simulink model "PhaseII_opalrt_NoProtection"  (Simulink 8.8)
settings: Solver=ode3  StartTime=0.0  StopTime=inf  FixedStep=Ts  RelTol=1e-5  EnableMultiTasking=on
PostLoadFcn:
  | %BESS ctrl
  | Kpf=0.005*3*12;
  | Kif=5*6;
  | 
  | Kpf1=0.005*3*12;
  | Kif1=5*6;
  | Kp_v=0.016*15*35;
  | Ki_v=12*25;
  | 
  | Kp_v1=0.016*15*35;
  | Ki_v1=12*25;
  | 
  | Vabc_B=12.47e3;
  | Vdc_ref=Vabc_B*2;
  | Kpwm=sqrt(2)*Vabc_B/Vdc_ref;
  | ZB=Vabc_B^2/1e6;
  | R=0.005*ZB;
  | Ibasefull=673/2*sqrt(2);
  | 
  | 
  | Ts_Control=1e-4;
  | ts=0.05;
  | delay=0.2;
  | offset=10e3;
  | t_plan=60;
  | t_monitor=.2;
  | t_mon=t_monitor;
  | scalingfactor=1;
  | x=0.5;
  | n=6;
  | %t_plan=1/15;
  | %t_monitor=10/900;
  | %t_mon=10/900;
  | 
  | %t_plan=1/5;
  | %t_monitor=10/300;
  | %t_mon=10/300;
  | %scalingfactor=1/300;
  | 
  | f0=60;
  | 
  | Pabc_B=1e6;
  | Iabc_B=Pabc_B*sqrt(2/3)/Vabc_B;  % pk value
  | Imax_1=2.5;
  | Ptrans_B=Pabc_B*200;
  | 
  | Vdc_ref=Vabc_B*2;
  | 
  | ZB=Vabc_B^2/Pabc_B;
  | L=0.1*ZB/2/pi/60;
  | R=0.1*ZB;
  | C=1/(4*pi^2*(2e3)^2*L);
  | 
  | LL=0.005*ZB/2/pi/60;
  | RR=0.005*ZB;
  | 
  | RC=0.02;
  | 
  | %%% Initial SOC %%%%
  | SOC_ini_BESS1=0.5;
  | ... (+223 lines)
InitFcn:
  | %BESS ctrl
  | Kpf=0.005*3*12;
  | Kif=5*6;
  | 
  | Kpf1=0.005*3*12;
  | Kif1=5*6;
  | Kp_v=0.016*15*35;
  | Ki_v=12*25;
  | 
  | Kp_v1=0.016*15*35;
  | Ki_v1=12*25;
  | 
  | Vabc_B=12.47e3;
  | Vdc_ref=Vabc_B*2;
  | Kpwm=sqrt(2)*Vabc_B/Vdc_ref;
  | ZB=Vabc_B^2/1e6;
  | R=0.005*ZB;
  | Ibasefull=673/2*sqrt(2);
  | 
  | 
  | Ts_Control=1e-4;
  | ts=0.05;
  | delay=0.2;
  | offset=10e3;
  | t_plan=60;
  | t_monitor=.2;
  | t_mon=t_monitor;
  | scalingfactor=1;
  | x=0.5;
  | n=6;
  | %t_plan=1/15;
  | %t_monitor=10/900;
  | %t_mon=10/900;
  | 
  | %t_plan=1/5;
  | %t_monitor=10/300;
  | %t_mon=10/300;
  | %scalingfactor=1/300;
  | 
  | f0=60;
  | 
  | Pabc_B=1e6;
  | Iabc_B=Pabc_B*sqrt(2/3)/Vabc_B;  % pk value
  | Imax_1=2.5;
  | Ptrans_B=Pabc_B*200;
  | 
  | Vdc_ref=Vabc_B*2;
  | 
  | ZB=Vabc_B^2/Pabc_B;
  | L=0.1*ZB/2/pi/60;
  | R=0.1*ZB;
  | C=1/(4*pi^2*(2e3)^2*L);
  | 
  | LL=0.005*ZB/2/pi/60;
  | RR=0.005*ZB;
  | 
  | RC=0.02;
  | 
  | %%% Initial SOC %%%%
  | SOC_ini_BESS1=0.5;
  | ... (+223 lines)
undefined symbols (not defined in the file): D1, Delta, DiscIntNeverNeededParam, Left, PG2ref, type, V
libraries: powerlib x220, powerlib_meascontrol x82, dspstat3 x54, dsparch4 x43, dspswit3 x24, simulink x19, simulink_extras x12, powerlib_extras x11, ssn_lib x7, artemis x6, rtlab x5, rtio_generic_dnp3 x5
(part 6 of 9)

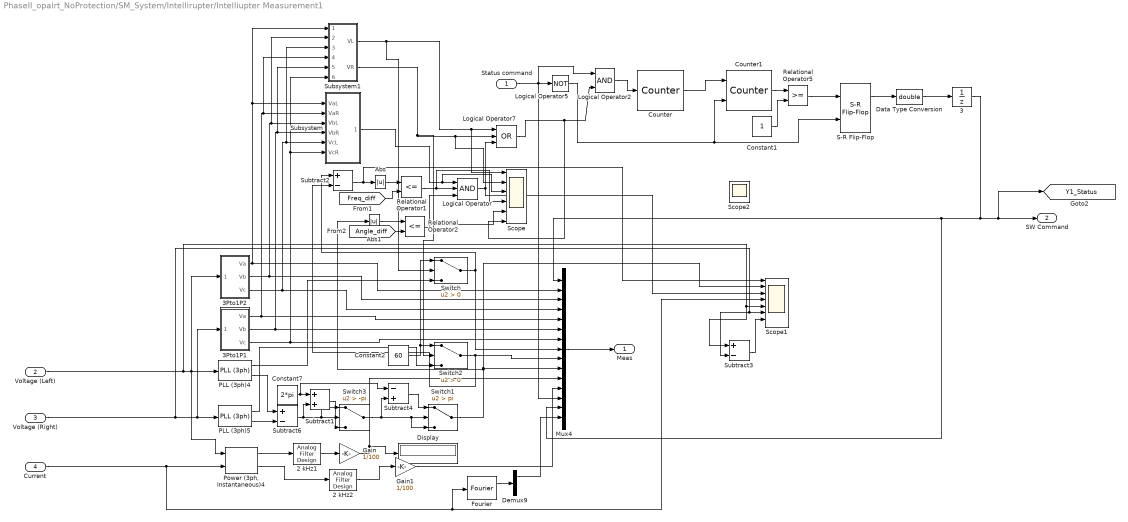
== system PhaseII_opalrt_NoProtection/SM_System/Intellirupter/Intelliupter Measurement1 ==
  Status command : Inport
  Voltage (Left) : Inport  Port=2
  Voltage (Right) : Inport  Port=3
  Current : Inport  Port=4
  "   3" : UnitDelay  SampleTime=Ts
  2 kHz1 : dsparch4/Analog Filter Design  method=Butterworth  filttype=Lowpass  N=2  Wlo=2*pi*5  Whi=80  Rp=2  Rs=40
  2 kHz2 : dsparch4/Analog Filter Design  method=Butterworth  filttype=Lowpass  N=2  Wlo=2*pi*5  Whi=80  Rp=2  Rs=40
  3Pto1P1 : Subsystem
  3Pto1P2 : Subsystem
  Abs : Abs
  Abs1 : Abs
  Constant1 : Constant
  Constant2 : Constant  Value=60
  Constant7 : Constant  Value=2*pi
  Counter : dspswit3/Counter  Direction=Up  CountEvent=Non-zero sample  CounterSize=User defined  MaxCount=10000  InitialCount=0  Output=Hit  HitValue=2000  ResetInput=off  SamplesPerFrame=1  Ts=1  CntDtype=double  HitDtype=Logical
  Counter1 : dspswit3/Counter  Direction=Up  CountEvent=Non-zero sample  CounterSize=User defined  MaxCount=255  InitialCount=0  Output=Count  HitValue=50  ResetInput=on  SamplesPerFrame=1  Ts=1  CntDtype=double  HitDtype=Logical
  Data Type Conversion : DataTypeConversion  OutDataTypeStr=double
  Demux9 : Demux  Outputs=3
  Display : Display
  Fourier : powerlib_meascontrol/Measurements/Fourier  Freq=60  n=1  InInit=[0, 0]  Ts=0
  Gain : Gain  Gain=1/100
  Gain1 : Gain  Gain=1/100
  Logical Operator : Logic  Inputs=3  AllPortsSameDT=off  OutDataTypeStr=boolean
  Logical Operator2 : Logic  AllPortsSameDT=off  OutDataTypeStr=boolean
  Logical Operator5 : Logic  Operator=NOT  AllPortsSameDT=off  OutDataTypeStr=boolean
  Logical Operator7 : Logic  Operator=OR  Inputs=3  AllPortsSameDT=off
  Mux4 : Mux  Inputs=15
  PLL (3ph)4 : powerlib_meascontrol/PLL/PLL (3ph)  Fmin=45  Par_Init=[0, 60]  ParK=[180, 3200, 1]  TcD=1e-4  MaxRateChangeFreq=12  FilterCutOffFreq=25  Ts=0  AGC=on
  PLL (3ph)5 : powerlib_meascontrol/PLL/PLL (3ph)  Fmin=45  Par_Init=[0, 60]  ParK=[180, 3200, 1]  TcD=1e-4  MaxRateChangeFreq=12  FilterCutOffFreq=25  Ts=0  AGC=on
  "Power (3ph, Instantaneous)4" : powerlib_meascontrol/Measurements/Power (3ph, Instantaneous)
  Relational Operator1 : RelationalOperator  Operator=<=  OutDataTypeStr=boolean  RndMeth=Simplest
  Relational Operator2 : RelationalOperator  Operator=<=  OutDataTypeStr=boolean  RndMeth=Simplest
  Relational Operator5 : RelationalOperator  OutDataTypeStr=boolean  RndMeth=Nearest
  S-R Flip-Flop : simulink_extras/Flip Flops/S-R Flip-Flop  initial_condition=0
  Scope : Scope  NumInputPorts=6
  Scope1 : Scope  NumInputPorts=8
  Scope2 : Scope  NumInputPorts=4
  Subsystem : Subsystem
  Subsystem1 : Subsystem
  Subtract1 : Sum
  Subtract2 : Sum  Inputs=+-
  Subtract3 : Sum  Inputs=+-
  Subtract4 : Sum  Inputs=-+
  Subtract6 : Sum  Inputs=+-
  Switch : Switch  Criteria=u2 > Threshold
  Switch1 : Switch  Criteria=u2 > Threshold  Threshold=pi
  Switch2 : Switch  Criteria=u2 > Threshold
  Switch3 : Switch  Criteria=u2 > Threshold  Threshold=-pi
  Meas : Outport
  SW Command : Outport  Port=2
  tag scope: Y1_Status=global
  wires:
  Logical Operator5/1 -> Counter1/2, S-R Flip-Flop/2
  Demux9/1 -> Mux4/15
  Fourier/1 -> Demux9/1
  Current/1 -> "Power (3ph, Instantaneous)4"/2, Scope1/4, Fourier/1
  Voltage (Left)/1 -> 3Pto1P2/1(Vabc), PLL (3ph)4/1, "Power (3ph, Instantaneous)4"/1, Scope1/5, Subtract3/1
  Subtract1/1 -> Switch3/3
  Subtract3/1 -> Scope1/7
  Constant7/1 -> Subtract4/1, Subtract1/1
  Subtract6/1 -> Switch3/2, Switch3/1, Subtract1/2
  Voltage (Right)/1 -> 3Pto1P1/1(Vabc), PLL (3ph)5/1, Scope1/6, Subtract3/2
  Subsystem1/2(VR) -> Switch2/2, Scope/2, Logical Operator7/2
  Subsystem1/1(VL) -> Switch/2, Scope/1, Logical Operator7/1
  Subsystem/1(Vdiff) -> Scope/3, Logical Operator/1
  Counter1/1 -> Relational Operator5/1
  Counter/1 -> Counter1/1
  Constant1/1 -> Relational Operator5/2
  Logical Operator2/1 -> Counter/1
  "Power (3ph, Instantaneous)4"/1 -> 2 kHz1/1
  PLL (3ph)4/1 -> Switch/3
  3Pto1P1/3(Vc) -> Mux4/7, Subsystem/6(VcR), Subsystem1/6(VcR)
  3Pto1P1/2(Vb) -> Mux4/6, Subsystem/4(VbR), Subsystem1/5(VbR)
  3Pto1P1/1(Va) -> Subsystem/2(VaR), Subsystem1/4(VaR), Mux4/5
  3Pto1P2/3(Vc) -> Mux4/4, Subsystem/5(VcL), Subsystem1/3(VcL)
  3Pto1P2/2(Vb) -> Subsystem/3(VbL), Subsystem1/2(VbL), Mux4/3
  3Pto1P2/1(Va) -> Mux4/2, Subsystem/1(VaL), Subsystem1/1(VaL)
  PLL (3ph)4/2 -> Subtract6/1
  Mux4/1 -> Meas/1
  PLL (3ph)5/2 -> Subtract6/2
  Relational Operator1/1 -> Scope/4, Logical Operator/2
  Relational Operator2/1 -> Scope/5, Logical Operator/3
  Subtract2/1 -> Abs/1, Scope1/1
  [Freq_diff] -> Relational Operator1/2
  [Angle_diff] -> Relational Operator2/2
  Logical Operator/1 -> Logical Operator7/3, Scope1/3
  Status command/1 -> Logical Operator2/1, Mux4/13, Logical Operator5/1
  Logical Operator7/1 -> Scope/6, Logical Operator2/2
  "Power (3ph, Instantaneous)4"/2 -> 2 kHz2/1
  "   3"/1 -> Mux4/1, Mux4/14, [Y1_Status], SW Command/1
  2 kHz1/1 -> Gain/1
  2 kHz2/1 -> Gain1/1
  Gain/1 -> Mux4/11, Display/1
  Gain1/1 -> Mux4/12
  S-R Flip-Flop/1 -> Data Type Conversion/1
  Relational Operator5/1 -> S-R Flip-Flop/1
  Data Type Conversion/1 -> "   3"/1
  Switch1/1 -> Scope1/2, Mux4/10, Abs1/1
  Subtract4/1 -> Switch1/1
  Switch3/1 -> Subtract4/2, Switch1/3, Switch1/2
  Abs/1 -> Relational Operator1/1
  Abs1/1 -> Relational Operator2/1
  Switch/1 -> Mux4/8, Subtract2/1
  Switch2/1 -> Subtract2/2, Mux4/9
  PLL (3ph)5/1 -> Switch2/3
  Constant2/1 -> Switch/1, Switch2/1

== system PhaseII_opalrt_NoProtection/SM_System/Intellirupter/Intelliupter Measurement2 ==
  Status command : Inport
  Voltage (Left) : Inport  Port=2
  Voltage (Right) : Inport  Port=3
  Current : Inport  Port=4
  "   3" : UnitDelay  SampleTime=Ts
  2 kHz1 : dsparch4/Analog Filter Design  method=Butterworth  filttype=Lowpass  N=2  Wlo=2*pi*5  Whi=80  Rp=2  Rs=40
  2 kHz2 : dsparch4/Analog Filter Design  method=Butterworth  filttype=Lowpass  N=2  Wlo=2*pi*5  Whi=80  Rp=2  Rs=40
  3Pto1P1 : Subsystem
  3Pto1P2 : Subsystem
  Abs : Abs
  Abs1 : Abs
  Constant1 : Constant
  Constant2 : Constant  Value=60
  Constant7 : Constant  Value=2*pi
  Counter : dspswit3/Counter  Direction=Up  CountEvent=Non-zero sample  CounterSize=User defined  MaxCount=10000  InitialCount=0  Output=Hit  HitValue=2000  ResetInput=off  SamplesPerFrame=1  Ts=1  CntDtype=double  HitDtype=Logical
  Counter1 : dspswit3/Counter  Direction=Up  CountEvent=Non-zero sample  CounterSize=User defined  MaxCount=255  InitialCount=0  Output=Count  HitValue=50  ResetInput=on  SamplesPerFrame=1  Ts=1  CntDtype=double  HitDtype=Logical
  Data Type Conversion : DataTypeConversion  OutDataTypeStr=double
  Demux9 : Demux  Outputs=3
  Display : Display
  Fourier : powerlib_meascontrol/Measurements/Fourier  Freq=60  n=1  InInit=[0, 0]  Ts=0
  Gain : Gain  Gain=1/100
  Gain1 : Gain  Gain=1/100
  Logical Operator : Logic  Inputs=3  AllPortsSameDT=off  OutDataTypeStr=boolean
  Logical Operator2 : Logic  AllPortsSameDT=off  OutDataTypeStr=boolean
  Logical Operator5 : Logic  Operator=NOT  AllPortsSameDT=off  OutDataTypeStr=boolean
  Logical Operator7 : Logic  Operator=OR  Inputs=3  AllPortsSameDT=off
  Mux4 : Mux  Inputs=15
  PLL (3ph)4 : powerlib_meascontrol/PLL/PLL (3ph)  Fmin=45  Par_Init=[0, 60]  ParK=[180, 3200, 1]  TcD=1e-4  MaxRateChangeFreq=12  FilterCutOffFreq=25  Ts=0  AGC=on
  PLL (3ph)5 : powerlib_meascontrol/PLL/PLL (3ph)  Fmin=45  Par_Init=[0, 60]  ParK=[180, 3200, 1]  TcD=1e-4  MaxRateChangeFreq=12  FilterCutOffFreq=25  Ts=0  AGC=on
  "Power (3ph, Instantaneous)4" : powerlib_meascontrol/Measurements/Power (3ph, Instantaneous)
  Relational Operator1 : RelationalOperator  Operator=<=  OutDataTypeStr=boolean  RndMeth=Simplest
  Relational Operator2 : RelationalOperator  Operator=<=  OutDataTypeStr=boolean  RndMeth=Simplest
  Relational Operator5 : RelationalOperator  OutDataTypeStr=boolean  RndMeth=Nearest
  S-R Flip-Flop : simulink_extras/Flip Flops/S-R Flip-Flop  initial_condition=0
  Scope1 : Scope  NumInputPorts=8
  Subsystem : Subsystem
  Subsystem1 : Subsystem
  Subtract1 : Sum
  Subtract2 : Sum  Inputs=+-
  Subtract3 : Sum  Inputs=+-
  Subtract4 : Sum  Inputs=-+
  Subtract6 : Sum  Inputs=+-
  Switch : Switch  Criteria=u2 > Threshold
  Switch1 : Switch  Criteria=u2 > Threshold  Threshold=pi
  Switch2 : Switch  Criteria=u2 > Threshold
  Switch3 : Switch  Criteria=u2 > Threshold  Threshold=-pi
  Meas : Outport
  SW Command : Outport  Port=2
  tag scope: Y2_Status=global
  wires:
  Logical Operator5/1 -> Counter1/2, S-R Flip-Flop/2
  "   3"/1 -> SW Command/1, [Y2_Status], Mux4/1, Mux4/14
  Demux9/1 -> Mux4/15
  Fourier/1 -> Demux9/1
  Current/1 -> "Power (3ph, Instantaneous)4"/2, Scope1/4, Fourier/1
  Voltage (Left)/1 -> 3Pto1P2/1(Vabc), PLL (3ph)4/1, "Power (3ph, Instantaneous)4"/1, Scope1/5, Subtract3/1
  Subtract1/1 -> Switch3/3
  Subtract3/1 -> Scope1/7
  Constant7/1 -> Subtract4/1, Subtract1/1
  Subtract6/1 -> Switch3/2, Switch3/1, Subtract1/2
  Voltage (Right)/1 -> 3Pto1P1/1(Vabc), PLL (3ph)5/1, Scope1/6, Subtract3/2
  Subsystem1/2(VR) -> Switch2/2, Logical Operator7/2
  Subsystem1/1(VL) -> Switch/2, Logical Operator7/1
  Subsystem/1(Vdiff) -> Logical Operator/1
  Counter1/1 -> Relational Operator5/1
  Counter/1 -> Counter1/1
  Constant1/1 -> Relational Operator5/2
  Logical Operator2/1 -> Counter/1
  "Power (3ph, Instantaneous)4"/1 -> 2 kHz1/1
  3Pto1P1/3(Vc) -> Mux4/7, Subsystem/6(VcR), Subsystem1/6(VcR)
  3Pto1P1/2(Vb) -> Mux4/6, Subsystem/4(VbR), Subsystem1/5(VbR)
  3Pto1P1/1(Va) -> Subsystem/2(VaR), Subsystem1/4(VaR), Mux4/5
  3Pto1P2/3(Vc) -> Mux4/4, Subsystem/5(VcL), Subsystem1/3(VcL)
  3Pto1P2/2(Vb) -> Subsystem/3(VbL), Subsystem1/2(VbL), Mux4/3
  3Pto1P2/1(Va) -> Mux4/2, Subsystem/1(VaL), Subsystem1/1(VaL)
  PLL (3ph)4/2 -> Subtract6/1
  Mux4/1 -> Meas/1
  PLL (3ph)5/2 -> Subtract6/2
  Relational Operator1/1 -> Logical Operator/2
  Relational Operator2/1 -> Logical Operator/3
  Subtract2/1 -> Abs/1, Scope1/1
  [Freq_diff] -> Relational Operator1/2
  [Angle_diff] -> Relational Operator2/2
  Logical Operator/1 -> Logical Operator7/3, Scope1/3
  Status command/1 -> Logical Operator2/1, Mux4/13, Logical Operator5/1
  Logical Operator7/1 -> Logical Operator2/2
  "Power (3ph, Instantaneous)4"/2 -> 2 kHz2/1
  2 kHz1/1 -> Gain/1
  2 kHz2/1 -> Gain1/1
  Gain/1 -> Mux4/11, Display/1
  Gain1/1 -> Mux4/12
  S-R Flip-Flop/1 -> Data Type Conversion/1
  Relational Operator5/1 -> S-R Flip-Flop/1
  Data Type Conversion/1 -> "   3"/1
  Switch1/1 -> Scope1/2, Mux4/10, Abs1/1
  Subtract4/1 -> Switch1/1
  Switch3/1 -> Subtract4/2, Switch1/3, Switch1/2
  Abs/1 -> Relational Operator1/1
  Abs1/1 -> Relational Operator2/1
  Switch/1 -> Subtract2/1, Mux4/8
  Switch2/1 -> Subtract2/2, Mux4/9
  PLL (3ph)4/1 -> Switch/3
  PLL (3ph)5/1 -> Switch2/3
  Constant2/1 -> Switch/1, Switch2/1

== system PhaseII_opalrt_NoProtection/SM_System/Intellirupter/Intelliupter Measurement3 ==
  Status command : Inport
  Voltage (Left) : Inport  Port=2
  Voltage (Right) : Inport  Port=3
  Current : Inport  Port=4
  "   3" : UnitDelay  SampleTime=Ts
  2 kHz1 : dsparch4/Analog Filter Design  method=Butterworth  filttype=Lowpass  N=2  Wlo=2*pi*5  Whi=80  Rp=2  Rs=40
  2 kHz2 : dsparch4/Analog Filter Design  method=Butterworth  filttype=Lowpass  N=2  Wlo=2*pi*5  Whi=80  Rp=2  Rs=40
  3Pto1P1 : Subsystem
  3Pto1P2 : Subsystem
  Abs : Abs
  Abs1 : Abs
  Constant1 : Constant
  Constant2 : Constant  Value=60
  Constant7 : Constant  Value=2*pi
  Counter : dspswit3/Counter  Direction=Up  CountEvent=Non-zero sample  CounterSize=User defined  MaxCount=10000  InitialCount=0  Output=Hit  HitValue=2000  ResetInput=off  SamplesPerFrame=1  Ts=1  CntDtype=double  HitDtype=Logical
  Counter1 : dspswit3/Counter  Direction=Up  CountEvent=Non-zero sample  CounterSize=User defined  MaxCount=255  InitialCount=0  Output=Count  HitValue=50  ResetInput=on  SamplesPerFrame=1  Ts=1  CntDtype=double  HitDtype=Logical
  Data Type Conversion : DataTypeConversion  OutDataTypeStr=double
  Demux9 : Demux  Outputs=3
  Display : Display
  Fourier : powerlib_meascontrol/Measurements/Fourier  Freq=60  n=1  InInit=[0, 0]  Ts=0
  Gain : Gain  Gain=1/100
  Gain1 : Gain  Gain=1/100
  Logical Operator : Logic  Inputs=3  AllPortsSameDT=off  OutDataTypeStr=boolean
  Logical Operator2 : Logic  AllPortsSameDT=off  OutDataTypeStr=boolean
  Logical Operator5 : Logic  Operator=NOT  AllPortsSameDT=off  OutDataTypeStr=boolean
  Logical Operator7 : Logic  Operator=OR  Inputs=3  AllPortsSameDT=off
  Mux4 : Mux  Inputs=15
  PLL (3ph)4 : powerlib_meascontrol/PLL/PLL (3ph)  Fmin=45  Par_Init=[0, 60]  ParK=[180, 3200, 1]  TcD=1e-4  MaxRateChangeFreq=12  FilterCutOffFreq=25  Ts=0  AGC=on
  PLL (3ph)5 : powerlib_meascontrol/PLL/PLL (3ph)  Fmin=45  Par_Init=[0, 60]  ParK=[180, 3200, 1]  TcD=1e-4  MaxRateChangeFreq=12  FilterCutOffFreq=25  Ts=0  AGC=on
  "Power (3ph, Instantaneous)4" : powerlib_meascontrol/Measurements/Power (3ph, Instantaneous)
  Relational Operator1 : RelationalOperator  Operator=<=  OutDataTypeStr=boolean  RndMeth=Simplest
  Relational Operator2 : RelationalOperator  Operator=<=  OutDataTypeStr=boolean  RndMeth=Simplest
  Relational Operator5 : RelationalOperator  OutDataTypeStr=boolean  RndMeth=Nearest
  S-R Flip-Flop : simulink_extras/Flip Flops/S-R Flip-Flop  initial_condition=0
  Scope1 : Scope  NumInputPorts=8
  Subsystem : Subsystem
  Subsystem1 : Subsystem
  Subtract1 : Sum
  Subtract2 : Sum  Inputs=+-
  Subtract3 : Sum  Inputs=+-
  Subtract4 : Sum  Inputs=-+
  Subtract6 : Sum  Inputs=+-
  Switch : Switch  Criteria=u2 > Threshold
  Switch1 : Switch  Criteria=u2 > Threshold  Threshold=pi
  Switch2 : Switch  Criteria=u2 > Threshold
  Switch3 : Switch  Criteria=u2 > Threshold  Threshold=-pi
  Meas : Outport
  SW Command : Outport  Port=2
  tag scope: Y3_Status=global
  wires:
  Logical Operator5/1 -> Counter1/2, S-R Flip-Flop/2
  "   3"/1 -> [Y3_Status], SW Command/1, Mux4/1, Mux4/14
  Demux9/1 -> Mux4/15
  Fourier/1 -> Demux9/1
  Current/1 -> "Power (3ph, Instantaneous)4"/2, Scope1/4, Fourier/1
  Voltage (Left)/1 -> 3Pto1P2/1(Vabc), PLL (3ph)4/1, "Power (3ph, Instantaneous)4"/1, Scope1/5, Subtract3/1
  Subtract1/1 -> Switch3/3
  Subtract3/1 -> Scope1/7
  Constant7/1 -> Subtract4/1, Subtract1/1
  Subtract6/1 -> Switch3/2, Switch3/1, Subtract1/2
  Voltage (Right)/1 -> 3Pto1P1/1(Vabc), PLL (3ph)5/1, Scope1/6, Subtract3/2
  Subsystem1/2(VR) -> Switch2/2, Logical Operator7/2
  Subsystem1/1(VL) -> Switch/2, Logical Operator7/1
  Subsystem/1(Vdiff) -> Logical Operator/1
  Counter1/1 -> Relational Operator5/1
  Counter/1 -> Counter1/1
  Constant1/1 -> Relational Operator5/2
  Logical Operator2/1 -> Counter/1
  "Power (3ph, Instantaneous)4"/1 -> 2 kHz1/1
  3Pto1P1/3(Vc) -> Mux4/7, Subsystem/6(VcR), Subsystem1/6(VcR)
  3Pto1P1/2(Vb) -> Mux4/6, Subsystem/4(VbR), Subsystem1/5(VbR)
  3Pto1P1/1(Va) -> Subsystem/2(VaR), Subsystem1/4(VaR), Mux4/5
  3Pto1P2/3(Vc) -> Mux4/4, Subsystem/5(VcL), Subsystem1/3(VcL)
  3Pto1P2/2(Vb) -> Subsystem/3(VbL), Subsystem1/2(VbL), Mux4/3
  3Pto1P2/1(Va) -> Mux4/2, Subsystem/1(VaL), Subsystem1/1(VaL)
  PLL (3ph)4/2 -> Subtract6/1
  Mux4/1 -> Meas/1
  PLL (3ph)5/2 -> Subtract6/2
  Relational Operator1/1 -> Logical Operator/2
  Relational Operator2/1 -> Logical Operator/3
  Subtract2/1 -> Abs/1, Scope1/1
  [Freq_diff] -> Relational Operator1/2
  [Angle_diff] -> Relational Operator2/2
  Logical Operator/1 -> Logical Operator7/3, Scope1/3
  Status command/1 -> Logical Operator2/1, Mux4/13, Logical Operator5/1
  Logical Operator7/1 -> Logical Operator2/2
  "Power (3ph, Instantaneous)4"/2 -> 2 kHz2/1
  2 kHz1/1 -> Gain/1
  2 kHz2/1 -> Gain1/1
  Gain/1 -> Mux4/11, Display/1
  Gain1/1 -> Mux4/12
  S-R Flip-Flop/1 -> Data Type Conversion/1
  Relational Operator5/1 -> S-R Flip-Flop/1
  Data Type Conversion/1 -> "   3"/1
  Switch1/1 -> Abs1/1, Scope1/2, Mux4/10
  Subtract4/1 -> Switch1/1
  Switch3/1 -> Subtract4/2, Switch1/3, Switch1/2
  Abs/1 -> Relational Operator1/1
  Abs1/1 -> Relational Operator2/1
  PLL (3ph)4/1 -> Switch/3
  PLL (3ph)5/1 -> Switch2/3
  Switch/1 -> Mux4/8, Subtract2/1
  Switch2/1 -> Subtract2/2, Mux4/9
  Constant2/1 -> Switch2/1, Switch/1

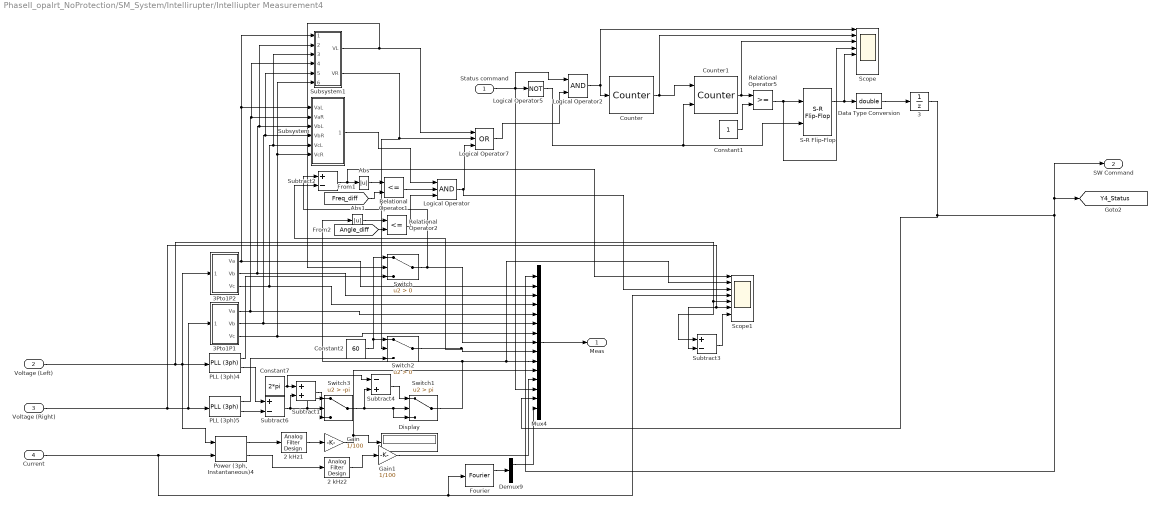
== system PhaseII_opalrt_NoProtection/SM_System/Intellirupter/Intelliupter Measurement4 ==
  Status command : Inport
  Voltage (Left) : Inport  Port=2
  Voltage (Right) : Inport  Port=3
  Current : Inport  Port=4
  "   3" : UnitDelay  SampleTime=Ts
  2 kHz1 : dsparch4/Analog Filter Design  method=Butterworth  filttype=Lowpass  N=2  Wlo=2*pi*5  Whi=80  Rp=2  Rs=40
  2 kHz2 : dsparch4/Analog Filter Design  method=Butterworth  filttype=Lowpass  N=2  Wlo=2*pi*5  Whi=80  Rp=2  Rs=40
  3Pto1P1 : Subsystem
  3Pto1P2 : Subsystem
  Abs : Abs
  Abs1 : Abs
  Constant1 : Constant
  Constant2 : Constant  Value=60
  Constant7 : Constant  Value=2*pi
  Counter : dspswit3/Counter  Direction=Up  CountEvent=Non-zero sample  CounterSize=User defined  MaxCount=10000  InitialCount=0  Output=Hit  HitValue=2000  ResetInput=off  SamplesPerFrame=1  Ts=1  CntDtype=double  HitDtype=Logical
  Counter1 : dspswit3/Counter  Direction=Up  CountEvent=Non-zero sample  CounterSize=User defined  MaxCount=255  InitialCount=0  Output=Count  HitValue=50  ResetInput=on  SamplesPerFrame=1  Ts=1  CntDtype=double  HitDtype=Logical
  Data Type Conversion : DataTypeConversion  OutDataTypeStr=double
  Demux9 : Demux  Outputs=3
  Display : Display
  Fourier : powerlib_meascontrol/Measurements/Fourier  Freq=60  n=1  InInit=[0, 0]  Ts=0
  Gain : Gain  Gain=1/100
  Gain1 : Gain  Gain=1/100
  Logical Operator : Logic  Inputs=3  AllPortsSameDT=off  OutDataTypeStr=boolean
  Logical Operator2 : Logic  AllPortsSameDT=off  OutDataTypeStr=boolean
  Logical Operator5 : Logic  Operator=NOT  AllPortsSameDT=off  OutDataTypeStr=boolean
  Logical Operator7 : Logic  Operator=OR  Inputs=3  AllPortsSameDT=off
  Mux4 : Mux  Inputs=15
  PLL (3ph)4 : powerlib_meascontrol/PLL/PLL (3ph)  Fmin=45  Par_Init=[0, 60]  ParK=[180, 3200, 1]  TcD=1e-4  MaxRateChangeFreq=12  FilterCutOffFreq=25  Ts=0  AGC=on
  PLL (3ph)5 : powerlib_meascontrol/PLL/PLL (3ph)  Fmin=45  Par_Init=[0, 60]  ParK=[180, 3200, 1]  TcD=1e-4  MaxRateChangeFreq=12  FilterCutOffFreq=25  Ts=0  AGC=on
  "Power (3ph, Instantaneous)4" : powerlib_meascontrol/Measurements/Power (3ph, Instantaneous)
  Relational Operator1 : RelationalOperator  Operator=<=  OutDataTypeStr=boolean  RndMeth=Simplest
  Relational Operator2 : RelationalOperator  Operator=<=  OutDataTypeStr=boolean  RndMeth=Simplest
  Relational Operator5 : RelationalOperator  OutDataTypeStr=boolean  RndMeth=Nearest
  S-R Flip-Flop : simulink_extras/Flip Flops/S-R Flip-Flop  initial_condition=0
  Scope : Scope  NumInputPorts=8
  Scope1 : Scope  NumInputPorts=8
  Subsystem : Subsystem
  Subsystem1 : Subsystem
  Subtract1 : Sum
  Subtract2 : Sum  Inputs=+-
  Subtract3 : Sum  Inputs=+-
  Subtract4 : Sum  Inputs=-+
  Subtract6 : Sum  Inputs=+-
  Switch : Switch  Criteria=u2 > Threshold
  Switch1 : Switch  Criteria=u2 > Threshold  Threshold=pi
  Switch2 : Switch  Criteria=u2 > Threshold
  Switch3 : Switch  Criteria=u2 > Threshold  Threshold=-pi
  Meas : Outport
  SW Command : Outport  Port=2
  tag scope: Y4_Status=global
  wires:
  Logical Operator5/1 -> Counter1/2, S-R Flip-Flop/2
  "   3"/1 -> Mux4/1, SW Command/1, [Y4_Status], Mux4/14
  Demux9/1 -> Mux4/15
  Fourier/1 -> Demux9/1
  Current/1 -> "Power (3ph, Instantaneous)4"/2, Scope1/4, Fourier/1
  Voltage (Left)/1 -> 3Pto1P2/1(Vabc), PLL (3ph)4/1, "Power (3ph, Instantaneous)4"/1, Scope1/5, Subtract3/1
  Subtract1/1 -> Switch3/3
  Subtract3/1 -> Scope1/7
  Constant7/1 -> Subtract4/1, Subtract1/1
  Subtract6/1 -> Switch3/2, Switch3/1, Subtract1/2
  Voltage (Right)/1 -> 3Pto1P1/1(Vabc), PLL (3ph)5/1, Scope1/6, Subtract3/2
  Subsystem1/2(VR) -> Switch2/2, Logical Operator7/2
  Subsystem1/1(VL) -> Switch/2, Logical Operator7/1
  Subsystem/1(Vdiff) -> Logical Operator/1
  Counter1/1 -> Relational Operator5/1, Scope/3
  Counter/1 -> Counter1/1, Scope/2
  Constant1/1 -> Relational Operator5/2
  Logical Operator2/1 -> Scope/1, Counter/1
  "Power (3ph, Instantaneous)4"/1 -> 2 kHz1/1
  3Pto1P1/3(Vc) -> Mux4/7, Subsystem/6(VcR), Subsystem1/6(VcR)
  3Pto1P1/2(Vb) -> Mux4/6, Subsystem/4(VbR), Subsystem1/5(VbR)
  3Pto1P1/1(Va) -> Subsystem/2(VaR), Subsystem1/4(VaR), Mux4/5
  3Pto1P2/3(Vc) -> Mux4/4, Subsystem/5(VcL), Subsystem1/3(VcL)
  3Pto1P2/2(Vb) -> Subsystem/3(VbL), Subsystem1/2(VbL), Mux4/3
  3Pto1P2/1(Va) -> Mux4/2, Subsystem/1(VaL), Subsystem1/1(VaL)
  PLL (3ph)4/2 -> Subtract6/1
  Mux4/1 -> Meas/1
  PLL (3ph)5/2 -> Subtract6/2
  Relational Operator1/1 -> Logical Operator/2
  Relational Operator2/1 -> Logical Operator/3
  Subtract2/1 -> Abs/1, Scope1/1
  [Freq_diff] -> Relational Operator1/2
  [Angle_diff] -> Relational Operator2/2
  Logical Operator/1 -> Logical Operator7/3, Scope1/3
  Status command/1 -> Logical Operator2/1, Mux4/13, Logical Operator5/1
  Logical Operator7/1 -> Logical Operator2/2
  "Power (3ph, Instantaneous)4"/2 -> 2 kHz2/1
  2 kHz1/1 -> Gain/1
  2 kHz2/1 -> Gain1/1
  Gain/1 -> Mux4/11, Display/1
  Gain1/1 -> Mux4/12
  S-R Flip-Flop/1 -> Data Type Conversion/1, Scope/5
  Relational Operator5/1 -> S-R Flip-Flop/1, Scope/4
  Data Type Conversion/1 -> "   3"/1
  Switch1/1 -> Scope1/2, Mux4/10, Abs1/1
  Subtract4/1 -> Switch1/1
  Switch3/1 -> Subtract4/2, Switch1/3, Switch1/2
  Abs/1 -> Relational Operator1/1
  Abs1/1 -> Relational Operator2/1
  Switch2/1 -> Subtract2/2, Mux4/9
  Switch/1 -> Mux4/8, Subtract2/1
  PLL (3ph)4/1 -> Switch/3
  PLL (3ph)5/1 -> Switch2/3
  Constant2/1 -> Switch/1, Switch2/1

== system PhaseII_opalrt_NoProtection/SM_System/Intellirupter/Intelliupter Measurement5 ==
  Status command : Inport
  Voltage (Left) : Inport  Port=2
  Voltage (Right) : Inport  Port=3
  Current : Inport  Port=4
  "   3" : UnitDelay  SampleTime=Ts
  2 kHz1 : dsparch4/Analog Filter Design  method=Butterworth  filttype=Lowpass  N=2  Wlo=2*pi*5  Whi=80  Rp=2  Rs=40
  2 kHz2 : dsparch4/Analog Filter Design  method=Butterworth  filttype=Lowpass  N=2  Wlo=2*pi*5  Whi=80  Rp=2  Rs=40
  3Pto1P1 : Subsystem
  3Pto1P2 : Subsystem
  Abs : Abs
  Abs1 : Abs
  Constant1 : Constant
  Constant2 : Constant  Value=60
  Constant7 : Constant  Value=2*pi
  Counter : dspswit3/Counter  Direction=Up  CountEvent=Non-zero sample  CounterSize=User defined  MaxCount=10000  InitialCount=0  Output=Hit  HitValue=2000  ResetInput=off  SamplesPerFrame=1  Ts=1  CntDtype=double  HitDtype=Logical
  Counter1 : dspswit3/Counter  Direction=Up  CountEvent=Non-zero sample  CounterSize=User defined  MaxCount=255  InitialCount=0  Output=Count  HitValue=50  ResetInput=on  SamplesPerFrame=1  Ts=1  CntDtype=double  HitDtype=Logical
  Data Type Conversion : DataTypeConversion  OutDataTypeStr=double
  Demux9 : Demux  Outputs=3
  Display : Display
  Fourier : powerlib_meascontrol/Measurements/Fourier  Freq=60  n=1  InInit=[0, 0]  Ts=0
  Gain : Gain  Gain=1/100
  Gain1 : Gain  Gain=1/100
  Logical Operator : Logic  Inputs=3  AllPortsSameDT=off  OutDataTypeStr=boolean
  Logical Operator2 : Logic  AllPortsSameDT=off  OutDataTypeStr=boolean
  Logical Operator5 : Logic  Operator=NOT  AllPortsSameDT=off  OutDataTypeStr=boolean
  Logical Operator7 : Logic  Operator=OR  Inputs=3  AllPortsSameDT=off
  Mux4 : Mux  Inputs=15
  PLL (3ph)4 : powerlib_meascontrol/PLL/PLL (3ph)  Fmin=45  Par_Init=[0, 60]  ParK=[180, 3200, 1]  TcD=1e-4  MaxRateChangeFreq=12  FilterCutOffFreq=25  Ts=0  AGC=on
  PLL (3ph)5 : powerlib_meascontrol/PLL/PLL (3ph)  Fmin=45  Par_Init=[0, 60]  ParK=[180, 3200, 1]  TcD=1e-4  MaxRateChangeFreq=12  FilterCutOffFreq=25  Ts=0  AGC=on
  "Power (3ph, Instantaneous)4" : powerlib_meascontrol/Measurements/Power (3ph, Instantaneous)
  Relational Operator1 : RelationalOperator  Operator=<=  OutDataTypeStr=boolean  RndMeth=Simplest
  Relational Operator2 : RelationalOperator  Operator=<=  OutDataTypeStr=boolean  RndMeth=Simplest
  Relational Operator5 : RelationalOperator  OutDataTypeStr=boolean  RndMeth=Nearest
  S-R Flip-Flop : simulink_extras/Flip Flops/S-R Flip-Flop  initial_condition=0
  Scope1 : Scope  NumInputPorts=8
  Subsystem : Subsystem
  Subsystem1 : Subsystem
  Subtract1 : Sum
  Subtract2 : Sum  Inputs=+-
  Subtract3 : Sum  Inputs=+-
  Subtract4 : Sum  Inputs=-+
  Subtract6 : Sum  Inputs=+-
  Switch : Switch  Criteria=u2 > Threshold
  Switch1 : Switch  Criteria=u2 > Threshold  Threshold=pi
  Switch2 : Switch  Criteria=u2 > Threshold
  Switch3 : Switch  Criteria=u2 > Threshold  Threshold=-pi
  Meas : Outport
  SW Command : Outport  Port=2
  tag scope: Y5_Status=global
  wires:
  Abs1/1 -> Relational Operator2/1
  Abs/1 -> Relational Operator1/1
  Switch3/1 -> Switch1/2, Switch1/3, Subtract4/2
  Subtract4/1 -> Switch1/1
  Switch1/1 -> Mux4/10, Scope1/2, Abs1/1
  Data Type Conversion/1 -> "   3"/1
  Relational Operator5/1 -> S-R Flip-Flop/1
  S-R Flip-Flop/1 -> Data Type Conversion/1
  Gain1/1 -> Mux4/12
  Gain/1 -> Display/1, Mux4/11
  2 kHz2/1 -> Gain1/1
  2 kHz1/1 -> Gain/1
  "Power (3ph, Instantaneous)4"/2 -> 2 kHz2/1
  Logical Operator7/1 -> Logical Operator2/2
  Status command/1 -> Logical Operator5/1, Mux4/13, Logical Operator2/1
  Logical Operator/1 -> Scope1/3, Logical Operator7/3
  [Angle_diff] -> Relational Operator2/2
  [Freq_diff] -> Relational Operator1/2
  Subtract2/1 -> Scope1/1, Abs/1
  Relational Operator2/1 -> Logical Operator/3
  Relational Operator1/1 -> Logical Operator/2
  PLL (3ph)5/2 -> Subtract6/2
  Mux4/1 -> Meas/1
  PLL (3ph)4/2 -> Subtract6/1
  3Pto1P2/1(Va) -> Subsystem1/1(VaL), Subsystem/1(VaL), Mux4/2
  3Pto1P2/2(Vb) -> Mux4/3, Subsystem1/2(VbL), Subsystem/3(VbL)
  3Pto1P2/3(Vc) -> Subsystem1/3(VcL), Subsystem/5(VcL), Mux4/4
  3Pto1P1/1(Va) -> Mux4/5, Subsystem1/4(VaR), Subsystem/2(VaR)
  3Pto1P1/2(Vb) -> Subsystem1/5(VbR), Subsystem/4(VbR), Mux4/6
  3Pto1P1/3(Vc) -> Subsystem1/6(VcR), Subsystem/6(VcR), Mux4/7
  "Power (3ph, Instantaneous)4"/1 -> 2 kHz1/1
  Logical Operator2/1 -> Counter/1
  Constant1/1 -> Relational Operator5/2
  Counter/1 -> Counter1/1
  Counter1/1 -> Relational Operator5/1
  Subsystem/1(Vdiff) -> Logical Operator/1
  Subsystem1/1(VL) -> Logical Operator7/1, Switch/2
  Subsystem1/2(VR) -> Switch2/2, Logical Operator7/2
  Voltage (Right)/1 -> Subtract3/2, Scope1/6, PLL (3ph)5/1, 3Pto1P1/1(Vabc)
  Subtract6/1 -> Subtract1/2, Switch3/1, Switch3/2
  Constant7/1 -> Subtract1/1, Subtract4/1
  Subtract3/1 -> Scope1/7
  Subtract1/1 -> Switch3/3
  Voltage (Left)/1 -> Subtract3/1, Scope1/5, "Power (3ph, Instantaneous)4"/1, PLL (3ph)4/1, 3Pto1P2/1(Vabc)
  Current/1 -> Fourier/1, Scope1/4, "Power (3ph, Instantaneous)4"/2
  Fourier/1 -> Demux9/1
  Demux9/1 -> Mux4/15
  "   3"/1 -> [Y5_Status], SW Command/1, Mux4/1, Mux4/14
  Logical Operator5/1 -> S-R Flip-Flop/2, Counter1/2
  PLL (3ph)4/1 -> Switch/3
  PLL (3ph)5/1 -> Switch2/3
  Switch/1 -> Subtract2/1, Mux4/8
  Switch2/1 -> Subtract2/2, Mux4/9
  Constant2/1 -> Switch2/1, Switch/1

== system PhaseII_opalrt_NoProtection/SM_System/Intellirupter/Intelliupter Measurement6 ==
  Status command : Inport
  Voltage (Left) : Inport  Port=2
  Voltage (Right) : Inport  Port=3
  Current : Inport  Port=4
  "   3" : UnitDelay  SampleTime=Ts
  2 kHz1 : dsparch4/Analog Filter Design  method=Butterworth  filttype=Lowpass  N=2  Wlo=2*pi*5  Whi=80  Rp=2  Rs=40
  2 kHz2 : dsparch4/Analog Filter Design  method=Butterworth  filttype=Lowpass  N=2  Wlo=2*pi*5  Whi=80  Rp=2  Rs=40
  3Pto1P1 : Subsystem
  3Pto1P2 : Subsystem
  Abs : Abs
  Abs1 : Abs
  Constant1 : Constant
  Constant2 : Constant  Value=60
  Constant7 : Constant  Value=2*pi
  Counter : dspswit3/Counter  Direction=Up  CountEvent=Non-zero sample  CounterSize=User defined  MaxCount=10000  InitialCount=0  Output=Hit  HitValue=2000  ResetInput=off  SamplesPerFrame=1  Ts=1  CntDtype=double  HitDtype=Logical
  Counter1 : dspswit3/Counter  Direction=Up  CountEvent=Non-zero sample  CounterSize=User defined  MaxCount=255  InitialCount=0  Output=Count  HitValue=50  ResetInput=on  SamplesPerFrame=1  Ts=1  CntDtype=double  HitDtype=Logical
  Data Type Conversion : DataTypeConversion  OutDataTypeStr=double
  Demux9 : Demux  Outputs=3
  Display : Display
  Fourier : powerlib_meascontrol/Measurements/Fourier  Freq=60  n=1  InInit=[0, 0]  Ts=0
  Gain : Gain  Gain=1/100
  Gain1 : Gain  Gain=1/100
  Logical Operator : Logic  Inputs=3  AllPortsSameDT=off  OutDataTypeStr=boolean
  Logical Operator2 : Logic  AllPortsSameDT=off  OutDataTypeStr=boolean
  Logical Operator5 : Logic  Operator=NOT  AllPortsSameDT=off  OutDataTypeStr=boolean
  Logical Operator7 : Logic  Operator=OR  Inputs=3  AllPortsSameDT=off
  Mux4 : Mux  Inputs=15
  PLL (3ph)4 : powerlib_meascontrol/PLL/PLL (3ph)  Fmin=45  Par_Init=[0, 60]  ParK=[180, 3200, 1]  TcD=1e-4  MaxRateChangeFreq=12  FilterCutOffFreq=25  Ts=0  AGC=on
  PLL (3ph)5 : powerlib_meascontrol/PLL/PLL (3ph)  Fmin=45  Par_Init=[0, 60]  ParK=[180, 3200, 1]  TcD=1e-4  MaxRateChangeFreq=12  FilterCutOffFreq=25  Ts=0  AGC=on
  "Power (3ph, Instantaneous)4" : powerlib_meascontrol/Measurements/Power (3ph, Instantaneous)
  Relational Operator1 : RelationalOperator  Operator=<=  OutDataTypeStr=boolean  RndMeth=Simplest
  Relational Operator2 : RelationalOperator  Operator=<=  OutDataTypeStr=boolean  RndMeth=Simplest
  Relational Operator5 : RelationalOperator  OutDataTypeStr=boolean  RndMeth=Nearest
  S-R Flip-Flop : simulink_extras/Flip Flops/S-R Flip-Flop  initial_condition=0
  Scope1 : Scope  NumInputPorts=8
  Subsystem : Subsystem
  Subsystem1 : Subsystem
  Subtract1 : Sum
  Subtract2 : Sum  Inputs=+-
  Subtract3 : Sum  Inputs=+-
  Subtract4 : Sum  Inputs=-+
  Subtract6 : Sum  Inputs=+-
  Switch : Switch  Criteria=u2 > Threshold
  Switch1 : Switch  Criteria=u2 > Threshold  Threshold=pi
  Switch2 : Switch  Criteria=u2 > Threshold
  Switch3 : Switch  Criteria=u2 > Threshold  Threshold=-pi
  Meas : Outport
  SW Command : Outport  Port=2
  tag scope: Y6_status=global
  wires:
  Logical Operator5/1 -> Counter1/2, S-R Flip-Flop/2
  "   3"/1 -> Mux4/1, Mux4/14, [Y6_status], SW Command/1
  Demux9/1 -> Mux4/15
  Fourier/1 -> Demux9/1
  Current/1 -> "Power (3ph, Instantaneous)4"/2, Scope1/4, Fourier/1
  Voltage (Left)/1 -> 3Pto1P2/1(Vabc), PLL (3ph)4/1, "Power (3ph, Instantaneous)4"/1, Scope1/5, Subtract3/1
  Subtract1/1 -> Switch3/3
  Subtract3/1 -> Scope1/7
  Constant7/1 -> Subtract4/1, Subtract1/1
  Subtract6/1 -> Switch3/2, Switch3/1, Subtract1/2
  Voltage (Right)/1 -> 3Pto1P1/1(Vabc), PLL (3ph)5/1, Scope1/6, Subtract3/2
  Subsystem1/2(VR) -> Logical Operator7/2, Switch2/2
  Subsystem1/1(VL) -> Switch/2, Logical Operator7/1
  Subsystem/1(Vdiff) -> Logical Operator/1
  Counter1/1 -> Relational Operator5/1
  Counter/1 -> Counter1/1
  Constant1/1 -> Relational Operator5/2
  Logical Operator2/1 -> Counter/1
  "Power (3ph, Instantaneous)4"/1 -> 2 kHz1/1
  3Pto1P1/3(Vc) -> Mux4/7, Subsystem/6(VcR), Subsystem1/6(VcR)
  3Pto1P1/2(Vb) -> Mux4/6, Subsystem/4(VbR), Subsystem1/5(VbR)
  3Pto1P1/1(Va) -> Subsystem/2(VaR), Subsystem1/4(VaR), Mux4/5
  3Pto1P2/3(Vc) -> Mux4/4, Subsystem/5(VcL), Subsystem1/3(VcL)
  3Pto1P2/2(Vb) -> Subsystem/3(VbL), Subsystem1/2(VbL), Mux4/3
  3Pto1P2/1(Va) -> Mux4/2, Subsystem/1(VaL), Subsystem1/1(VaL)
  PLL (3ph)4/2 -> Subtract6/1
  Mux4/1 -> Meas/1
  PLL (3ph)5/2 -> Subtract6/2
  Relational Operator1/1 -> Logical Operator/2
  Relational Operator2/1 -> Logical Operator/3
  Subtract2/1 -> Abs/1, Scope1/1
  [Freq_diff] -> Relational Operator1/2
  [Angle_diff] -> Relational Operator2/2
  Logical Operator/1 -> Logical Operator7/3, Scope1/3
  Status command/1 -> Logical Operator2/1, Mux4/13, Logical Operator5/1
  Logical Operator7/1 -> Logical Operator2/2
  "Power (3ph, Instantaneous)4"/2 -> 2 kHz2/1
  2 kHz1/1 -> Gain/1
  2 kHz2/1 -> Gain1/1
  Gain/1 -> Mux4/11, Display/1
  Gain1/1 -> Mux4/12
  S-R Flip-Flop/1 -> Data Type Conversion/1
  Relational Operator5/1 -> S-R Flip-Flop/1
  Data Type Conversion/1 -> "   3"/1
  Switch1/1 -> Abs1/1, Scope1/2, Mux4/10
  Subtract4/1 -> Switch1/1
  Switch3/1 -> Subtract4/2, Switch1/3, Switch1/2
  Abs/1 -> Relational Operator1/1
  Abs1/1 -> Relational Operator2/1
  Switch/1 -> Subtract2/1, Mux4/8
  Switch2/1 -> Subtract2/2, Mux4/9
  PLL (3ph)5/1 -> Switch2/3
  PLL (3ph)4/1 -> Switch/3
  Constant2/1 -> Switch2/1, Switch/1

== system PhaseII_opalrt_NoProtection/SM_System/Intellirupter/Intelliupter Measurement7 ==
  Status command : Inport
  Voltage (Left) : Inport  Port=2
  Voltage (Right) : Inport  Port=3
  Current : Inport  Port=4
  "   3" : UnitDelay  SampleTime=Ts
  2 kHz1 : dsparch4/Analog Filter Design  method=Butterworth  filttype=Lowpass  N=2  Wlo=2*pi*5  Whi=80  Rp=2  Rs=40
  2 kHz2 : dsparch4/Analog Filter Design  method=Butterworth  filttype=Lowpass  N=2  Wlo=2*pi*5  Whi=80  Rp=2  Rs=40
  3Pto1P1 : Subsystem
  3Pto1P2 : Subsystem
  Abs : Abs
  Abs1 : Abs
  Constant1 : Constant
  Constant2 : Constant  Value=60
  Constant7 : Constant  Value=2*pi
  Counter : dspswit3/Counter  Direction=Up  CountEvent=Non-zero sample  CounterSize=User defined  MaxCount=10000  InitialCount=0  Output=Hit  HitValue=2000  ResetInput=off  SamplesPerFrame=1  Ts=1  CntDtype=double  HitDtype=Logical
  Counter1 : dspswit3/Counter  Direction=Up  CountEvent=Non-zero sample  CounterSize=User defined  MaxCount=255  InitialCount=0  Output=Count  HitValue=50  ResetInput=on  SamplesPerFrame=1  Ts=1  CntDtype=double  HitDtype=Logical
  Data Type Conversion : DataTypeConversion  OutDataTypeStr=double
  Demux9 : Demux  Outputs=3
  Display : Display
  Fourier : powerlib_meascontrol/Measurements/Fourier  Freq=60  n=1  InInit=[0, 0]  Ts=0
  Gain : Gain  Gain=1/100
  Gain1 : Gain  Gain=1/100
  Logical Operator : Logic  Inputs=3  AllPortsSameDT=off  OutDataTypeStr=boolean
  Logical Operator2 : Logic  AllPortsSameDT=off  OutDataTypeStr=boolean
  Logical Operator5 : Logic  Operator=NOT  AllPortsSameDT=off  OutDataTypeStr=boolean
  Logical Operator7 : Logic  Operator=OR  Inputs=3  AllPortsSameDT=off
  Mux4 : Mux  Inputs=15
  PLL (3ph)4 : powerlib_meascontrol/PLL/PLL (3ph)  Fmin=45  Par_Init=[0, 60]  ParK=[180, 3200, 1]  TcD=1e-4  MaxRateChangeFreq=12  FilterCutOffFreq=25  Ts=0  AGC=on
  PLL (3ph)5 : powerlib_meascontrol/PLL/PLL (3ph)  Fmin=45  Par_Init=[0, 60]  ParK=[180, 3200, 1]  TcD=1e-4  MaxRateChangeFreq=12  FilterCutOffFreq=25  Ts=0  AGC=on
  "Power (3ph, Instantaneous)4" : powerlib_meascontrol/Measurements/Power (3ph, Instantaneous)
  Relational Operator1 : RelationalOperator  Operator=<=  OutDataTypeStr=boolean  RndMeth=Simplest
  Relational Operator2 : RelationalOperator  Operator=<=  OutDataTypeStr=boolean  RndMeth=Simplest
  Relational Operator5 : RelationalOperator  OutDataTypeStr=boolean  RndMeth=Nearest
  S-R Flip-Flop : simulink_extras/Flip Flops/S-R Flip-Flop  initial_condition=0
  Scope1 : Scope  NumInputPorts=8
  Subsystem : Subsystem
  Subsystem1 : Subsystem
  Subtract1 : Sum
  Subtract2 : Sum  Inputs=+-
  Subtract3 : Sum  Inputs=+-
  Subtract4 : Sum  Inputs=-+
  Subtract6 : Sum  Inputs=+-
  Switch : Switch  Criteria=u2 > Threshold
  Switch1 : Switch  Criteria=u2 > Threshold  Threshold=pi
  Switch2 : Switch  Criteria=u2 > Threshold
  Switch3 : Switch  Criteria=u2 > Threshold  Threshold=-pi
  Meas : Outport
  SW Command : Outport  Port=2
  tag scope: Y7_Status=global
  wires:
  Abs1/1 -> Relational Operator2/1
  Abs/1 -> Relational Operator1/1
  Switch3/1 -> Switch1/2, Switch1/3, Subtract4/2
  Subtract4/1 -> Switch1/1
  Switch1/1 -> Mux4/10, Scope1/2, Abs1/1
  Data Type Conversion/1 -> "   3"/1
  Relational Operator5/1 -> S-R Flip-Flop/1
  S-R Flip-Flop/1 -> Data Type Conversion/1
  Gain1/1 -> Mux4/12
  Gain/1 -> Display/1, Mux4/11
  2 kHz2/1 -> Gain1/1
  2 kHz1/1 -> Gain/1
  "Power (3ph, Instantaneous)4"/2 -> 2 kHz2/1
  Logical Operator7/1 -> Logical Operator2/2
  Status command/1 -> Logical Operator5/1, Mux4/13, Logical Operator2/1
  Logical Operator/1 -> Scope1/3, Logical Operator7/3
  [Angle_diff] -> Relational Operator2/2
  [Freq_diff] -> Relational Operator1/2
  Subtract2/1 -> Scope1/1, Abs/1
  Relational Operator2/1 -> Logical Operator/3
  Relational Operator1/1 -> Logical Operator/2
  PLL (3ph)5/2 -> Subtract6/2
  Mux4/1 -> Meas/1
  PLL (3ph)4/2 -> Subtract6/1
  3Pto1P2/1(Va) -> Subsystem1/1(VaL), Subsystem/1(VaL), Mux4/2
  3Pto1P2/2(Vb) -> Mux4/3, Subsystem1/2(VbL), Subsystem/3(VbL)
  3Pto1P2/3(Vc) -> Subsystem1/3(VcL), Subsystem/5(VcL), Mux4/4
  3Pto1P1/1(Va) -> Mux4/5, Subsystem1/4(VaR), Subsystem/2(VaR)
  3Pto1P1/2(Vb) -> Subsystem1/5(VbR), Subsystem/4(VbR), Mux4/6
  3Pto1P1/3(Vc) -> Subsystem1/6(VcR), Subsystem/6(VcR), Mux4/7
  "Power (3ph, Instantaneous)4"/1 -> 2 kHz1/1
  Logical Operator2/1 -> Counter/1
  Constant1/1 -> Relational Operator5/2
  Counter/1 -> Counter1/1
  Counter1/1 -> Relational Operator5/1
  Subsystem/1(Vdiff) -> Logical Operator/1
  Subsystem1/1(VL) -> Logical Operator7/1, Switch/2
  Subsystem1/2(VR) -> Logical Operator7/2, Switch2/2
  Voltage (Right)/1 -> Subtract3/2, Scope1/6, PLL (3ph)5/1, 3Pto1P1/1(Vabc)
  Subtract6/1 -> Subtract1/2, Switch3/1, Switch3/2
  Constant7/1 -> Subtract1/1, Subtract4/1
  Subtract3/1 -> Scope1/7
  Subtract1/1 -> Switch3/3
  Voltage (Left)/1 -> Subtract3/1, Scope1/5, "Power (3ph, Instantaneous)4"/1, PLL (3ph)4/1, 3Pto1P2/1(Vabc)
  Current/1 -> Fourier/1, Scope1/4, "Power (3ph, Instantaneous)4"/2
  Fourier/1 -> Demux9/1
  Demux9/1 -> Mux4/15
  "   3"/1 -> [Y7_Status], SW Command/1, Mux4/14, Mux4/1
  Logical Operator5/1 -> S-R Flip-Flop/2, Counter1/2
  Switch2/1 -> Subtract2/2, Mux4/9
  Switch/1 -> Subtract2/1, Mux4/8
  PLL (3ph)5/1 -> Switch2/3
  PLL (3ph)4/1 -> Switch/3
  Constant2/1 -> Switch/1, Switch2/1

== system PhaseII_opalrt_NoProtection/SM_System/Intellirupter/Intelliupter Measurement8 ==
  Status command : Inport
  Voltage (Left) : Inport  Port=2
  Voltage (Right) : Inport  Port=3
  Current : Inport  Port=4
  "   3" : UnitDelay  SampleTime=Ts
  2 kHz1 : dsparch4/Analog Filter Design  method=Butterworth  filttype=Lowpass  N=2  Wlo=2*pi*5  Whi=80  Rp=2  Rs=40
  2 kHz2 : dsparch4/Analog Filter Design  method=Butterworth  filttype=Lowpass  N=2  Wlo=2*pi*5  Whi=80  Rp=2  Rs=40
  3Pto1P1 : Subsystem
  3Pto1P2 : Subsystem
  Abs : Abs
  Abs1 : Abs
  Constant1 : Constant
  Constant2 : Constant  Value=60
  Constant7 : Constant  Value=2*pi
  Counter : dspswit3/Counter  Direction=Up  CountEvent=Non-zero sample  CounterSize=User defined  MaxCount=10000  InitialCount=0  Output=Hit  HitValue=2000  ResetInput=off  SamplesPerFrame=1  Ts=1  CntDtype=double  HitDtype=Logical
  Counter1 : dspswit3/Counter  Direction=Up  CountEvent=Non-zero sample  CounterSize=User defined  MaxCount=255  InitialCount=0  Output=Count  HitValue=50  ResetInput=on  SamplesPerFrame=1  Ts=1  CntDtype=double  HitDtype=Logical
  Data Type Conversion : DataTypeConversion  OutDataTypeStr=double
  Demux9 : Demux  Outputs=3
  Display : Display
  Fourier : powerlib_meascontrol/Measurements/Fourier  Freq=60  n=1  InInit=[0, 0]  Ts=0
  Gain : Gain  Gain=1/100
  Gain1 : Gain  Gain=1/100
  Logical Operator : Logic  Inputs=3  AllPortsSameDT=off  OutDataTypeStr=boolean
  Logical Operator2 : Logic  AllPortsSameDT=off  OutDataTypeStr=boolean
  Logical Operator5 : Logic  Operator=NOT  AllPortsSameDT=off  OutDataTypeStr=boolean
  Logical Operator7 : Logic  Operator=OR  Inputs=3  AllPortsSameDT=off
  Mux4 : Mux  Inputs=15
  PLL (3ph)4 : powerlib_meascontrol/PLL/PLL (3ph)  Fmin=45  Par_Init=[0, 60]  ParK=[180, 3200, 1]  TcD=1e-4  MaxRateChangeFreq=12  FilterCutOffFreq=25  Ts=0  AGC=on
  PLL (3ph)5 : powerlib_meascontrol/PLL/PLL (3ph)  Fmin=45  Par_Init=[0, 60]  ParK=[180, 3200, 1]  TcD=1e-4  MaxRateChangeFreq=12  FilterCutOffFreq=25  Ts=0  AGC=on
  "Power (3ph, Instantaneous)4" : powerlib_meascontrol/Measurements/Power (3ph, Instantaneous)
  Relational Operator1 : RelationalOperator  Operator=<=  OutDataTypeStr=boolean  RndMeth=Simplest
  Relational Operator2 : RelationalOperator  Operator=<=  OutDataTypeStr=boolean  RndMeth=Simplest
  Relational Operator5 : RelationalOperator  OutDataTypeStr=boolean  RndMeth=Nearest
  S-R Flip-Flop : simulink_extras/Flip Flops/S-R Flip-Flop  initial_condition=0
  Scope1 : Scope  NumInputPorts=8
  Subsystem : Subsystem
  Subsystem1 : Subsystem
  Subtract1 : Sum
  Subtract2 : Sum  Inputs=+-
  Subtract3 : Sum  Inputs=+-
  Subtract4 : Sum  Inputs=-+
  Subtract6 : Sum  Inputs=+-
  Switch : Switch  Criteria=u2 > Threshold
  Switch1 : Switch  Criteria=u2 > Threshold  Threshold=pi
  Switch2 : Switch  Criteria=u2 > Threshold
  Switch3 : Switch  Criteria=u2 > Threshold  Threshold=-pi
  Meas : Outport
  SW Command : Outport  Port=2
  tag scope: Y8_Status=global
  wires:
  Logical Operator5/1 -> Counter1/2, S-R Flip-Flop/2
  "   3"/1 -> SW Command/1, [Y8_Status], Mux4/1, Mux4/14
  Demux9/1 -> Mux4/15
  Fourier/1 -> Demux9/1
  Current/1 -> "Power (3ph, Instantaneous)4"/2, Scope1/4, Fourier/1
  Voltage (Left)/1 -> 3Pto1P2/1(Vabc), PLL (3ph)4/1, "Power (3ph, Instantaneous)4"/1, Scope1/5, Subtract3/1
  Subtract1/1 -> Switch3/3
  Subtract3/1 -> Scope1/7
  Constant7/1 -> Subtract4/1, Subtract1/1
  Subtract6/1 -> Switch3/2, Switch3/1, Subtract1/2
  Voltage (Right)/1 -> 3Pto1P1/1(Vabc), PLL (3ph)5/1, Scope1/6, Subtract3/2
  Subsystem1/1(VL) -> Switch/2, Logical Operator7/1
  Subsystem/1(Vdiff) -> Logical Operator/1
  Counter1/1 -> Relational Operator5/1
  Counter/1 -> Counter1/1
  Constant1/1 -> Relational Operator5/2
  Logical Operator2/1 -> Counter/1
  "Power (3ph, Instantaneous)4"/1 -> 2 kHz1/1
  3Pto1P1/3(Vc) -> Mux4/7, Subsystem/6(VcR), Subsystem1/6(VcR)
  3Pto1P1/2(Vb) -> Mux4/6, Subsystem/4(VbR), Subsystem1/5(VbR)
  3Pto1P1/1(Va) -> Subsystem/2(VaR), Subsystem1/4(VaR), Mux4/5
  3Pto1P2/3(Vc) -> Mux4/4, Subsystem/5(VcL), Subsystem1/3(VcL)
  3Pto1P2/2(Vb) -> Subsystem/3(VbL), Subsystem1/2(VbL), Mux4/3
  3Pto1P2/1(Va) -> Mux4/2, Subsystem/1(VaL), Subsystem1/1(VaL)
  PLL (3ph)4/2 -> Subtract6/1
  Mux4/1 -> Meas/1
  PLL (3ph)5/2 -> Subtract6/2
  Relational Operator1/1 -> Logical Operator/2
  Relational Operator2/1 -> Logical Operator/3
  Subtract2/1 -> Abs/1, Scope1/1
  [Freq_diff] -> Relational Operator1/2
  [Angle_diff] -> Relational Operator2/2
  Logical Operator/1 -> Logical Operator7/3, Scope1/3
  Status command/1 -> Logical Operator2/1, Mux4/13, Logical Operator5/1
  Logical Operator7/1 -> Logical Operator2/2
  "Power (3ph, Instantaneous)4"/2 -> 2 kHz2/1
  2 kHz1/1 -> Gain/1
  2 kHz2/1 -> Gain1/1
  Gain/1 -> Mux4/11, Display/1
  Gain1/1 -> Mux4/12
  S-R Flip-Flop/1 -> Data Type Conversion/1
  Relational Operator5/1 -> S-R Flip-Flop/1
  Data Type Conversion/1 -> "   3"/1
  Switch1/1 -> Scope1/2, Mux4/10, Abs1/1
  Subtract4/1 -> Switch1/1
  Switch3/1 -> Subtract4/2, Switch1/3, Switch1/2
  Abs/1 -> Relational Operator1/1
  Abs1/1 -> Relational Operator2/1
  Switch2/1 -> Subtract2/2, Mux4/9
  Switch/1 -> Subtract2/1, Mux4/8
  Subsystem1/2(VR) -> Switch2/2, Logical Operator7/2
  Constant2/1 -> Switch/1, Switch2/1
  PLL (3ph)5/1 -> Switch2/3
  PLL (3ph)4/1 -> Switch/3

== system PhaseII_opalrt_NoProtection/SM_System/Subsystem/Fault ==
  In7 : Inport
  Breaker : powerlib/Elements/Breaker  InitialState=0  SwitchingTimes="[1/60  5/60]"  External=on  BreakerResistance=0.001  SnubberResistance=1e6  SnubberCapacitance=inf  Measurements=None  MoreParameters=on  NoBreakLoop=off
  Breaker1 : powerlib/Elements/Breaker  InitialState=0  SwitchingTimes="[1/60  5/60]"  External=on  BreakerResistance=0.001  SnubberResistance=1e6  SnubberCapacitance=inf  Measurements=None  MoreParameters=on  NoBreakLoop=off
  Breaker2 : powerlib/Elements/Breaker  InitialState=0  SwitchingTimes="[1/60  5/60]"  External=on  BreakerResistance=0.001  SnubberResistance=1e6  SnubberCapacitance=inf  Measurements=None  MoreParameters=on  NoBreakLoop=off
  In1 : PMIOPort  Port=1  Side=Left
  In2 : PMIOPort  Port=2  Side=Right
  In3 : PMIOPort  Port=3  Side=Left
  In4 : PMIOPort  Port=4  Side=Right
  In5 : PMIOPort  Port=5  Side=Left
  In6 : PMIOPort  Port=6  Side=Right
  wires:
  In7/1 -> Breaker/1, Breaker2/1, Breaker1/1
  connections:
  Breaker/LConn1 -- In1/RConn1
  Breaker/RConn1 -- In2/RConn1
  Breaker1/LConn1 -- In3/RConn1
  Breaker1/RConn1 -- In4/RConn1
  Breaker2/RConn1 -- In6/RConn1
  Breaker2/LConn1 -- In5/RConn1

== system PhaseII_opalrt_NoProtection/SM_System/Subsystem1/Fault ==
  In7 : Inport
  Breaker : powerlib/Elements/Breaker  InitialState=0  SwitchingTimes="[1/60  5/60]"  External=on  BreakerResistance=0.001  SnubberResistance=1e6  SnubberCapacitance=inf  Measurements=None  MoreParameters=on  NoBreakLoop=off
  Breaker1 : powerlib/Elements/Breaker  InitialState=0  SwitchingTimes="[1/60  5/60]"  External=on  BreakerResistance=0.001  SnubberResistance=1e6  SnubberCapacitance=inf  Measurements=None  MoreParameters=on  NoBreakLoop=off
  Breaker2 : powerlib/Elements/Breaker  InitialState=0  SwitchingTimes="[1/60  5/60]"  External=on  BreakerResistance=0.001  SnubberResistance=1e6  SnubberCapacitance=inf  Measurements=None  MoreParameters=on  NoBreakLoop=off
  In1 : PMIOPort  Port=1  Side=Left
  In2 : PMIOPort  Port=2  Side=Right
  In3 : PMIOPort  Port=3  Side=Left
  In4 : PMIOPort  Port=4  Side=Right
  In5 : PMIOPort  Port=5  Side=Left
  In6 : PMIOPort  Port=6  Side=Right
  wires:
  In7/1 -> Breaker1/1, Breaker2/1, Breaker/1
  connections:
  Breaker2/LConn1 -- In5/RConn1
  Breaker2/RConn1 -- In6/RConn1
  Breaker1/RConn1 -- In4/RConn1
  Breaker1/LConn1 -- In3/RConn1
  Breaker/RConn1 -- In2/RConn1
  Breaker/LConn1 -- In1/RConn1

== system PhaseII_opalrt_NoProtection/SM_System/Subsystem2/Fault ==
  In7 : Inport
  Breaker : powerlib/Elements/Breaker  InitialState=0  SwitchingTimes="[1/60  5/60]"  External=on  BreakerResistance=0.001  SnubberResistance=1e6  SnubberCapacitance=inf  Measurements=None  MoreParameters=on  NoBreakLoop=off
  Breaker1 : powerlib/Elements/Breaker  InitialState=0  SwitchingTimes="[1/60  5/60]"  External=on  BreakerResistance=0.001  SnubberResistance=1e6  SnubberCapacitance=inf  Measurements=None  MoreParameters=on  NoBreakLoop=off
  Breaker2 : powerlib/Elements/Breaker  InitialState=0  SwitchingTimes="[1/60  5/60]"  External=on  BreakerResistance=0.001  SnubberResistance=1e6  SnubberCapacitance=inf  Measurements=None  MoreParameters=on  NoBreakLoop=off
  In1 : PMIOPort  Port=1  Side=Left
  In2 : PMIOPort  Port=2  Side=Right
  In3 : PMIOPort  Port=3  Side=Left
  In4 : PMIOPort  Port=4  Side=Right
  In5 : PMIOPort  Port=5  Side=Left
  In6 : PMIOPort  Port=6  Side=Right
  wires:
  In7/1 -> Breaker/1, Breaker2/1, Breaker1/1
  connections:
  Breaker/LConn1 -- In1/RConn1
  Breaker/RConn1 -- In2/RConn1
  Breaker1/LConn1 -- In3/RConn1
  Breaker1/RConn1 -- In4/RConn1
  Breaker2/RConn1 -- In6/RConn1
  Breaker2/LConn1 -- In5/RConn1
